simulink library "telem_conversion_lib"  (R2014b)
settings: Solver=ode45  StartTime=0.0  StopTime=10.0  RelTol=1e-3
undefined symbols (not defined in the file or in its folder): ini_moon_rotation_rate
libraries: util_quat_lib x11, util_frame_rotation_lib x4, util_common_lib x4, util_info_lib x1
settings Model: Creator=escrane  LastModifiedBy=mstewart

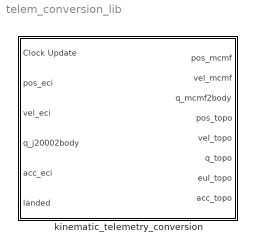
== system telem_conversion_lib ==
  kinematic_telemetry_conversion : Subsystem

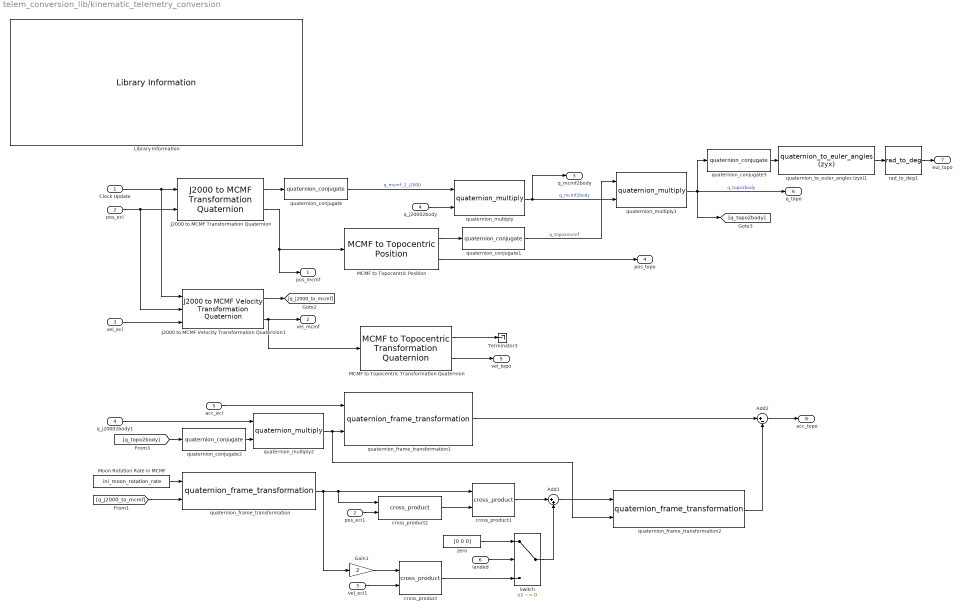
== system telem_conversion_lib/kinematic_telemetry_conversion ==
  Clock Update : Inport
  pos_eci : Inport  Port=2
  vel_eci : Inport  Port=3
  q_j20002body : Inport  Port=4
  acc_eci : Inport  Port=5
  landed : Inport  Port=6
  Add1 : Sum  Inputs=|++
  Add2 : Sum  Inputs=|+-
  Gain1 : Gain  Gain=2
  J2000 to MCMF Transformation Quaternion : util_frame_rotation_lib/J2000 to MCMF  Transformation Quaternion  SystemSampleTime=-1
  J2000 to MCMF Velocity Transformation Quaternion1 : util_frame_rotation_lib/J2000 to MCMF Velocity Transformation Quaternion  SystemSampleTime=-1
  Library Information : util_info_lib/Library Information  owner='NONE'
  MCMF to Topocentric Position : util_frame_rotation_lib/MCMF to Topocentric  Position  SystemSampleTime=-1
  MCMF to Topocentric Transformation Quaternion : util_frame_rotation_lib/MCMF to Topocentric  Transformation Quaternion  SystemSampleTime=-1
  Moon Rotation Rate in MCMF : Constant  Value=ini_moon_rotation_rate
  Switch : Switch  Criteria=u2 ~= 0
  Terminator3 : Terminator
  cross_product : util_common_lib/cross_product  SystemSampleTime=-1
  cross_product1 : util_common_lib/cross_product  SystemSampleTime=-1
  cross_product2 : util_common_lib/cross_product  SystemSampleTime=-1
  pos_eci1 : InportShadow  Port=2
  q_j20002body1 : InportShadow  Port=4
  quaternion_conjugate{,1..3} (4 alike) : util_quat_lib/quaternion_conjugate  SystemSampleTime=-1
  quaternion_frame_transformation : util_quat_lib/quaternion_frame_transformation  SystemSampleTime=-1
  quaternion_frame_transformation1 : util_quat_lib/quaternion_frame_transformation  SystemSampleTime=-1
  quaternion_frame_transformation2 : util_quat_lib/quaternion_frame_transformation  SystemSampleTime=-1
  quaternion_multiply : util_quat_lib/quaternion_multiply  SystemSampleTime=-1
  quaternion_multiply1 : util_quat_lib/quaternion_multiply  SystemSampleTime=-1
  quaternion_multiply2 : util_quat_lib/quaternion_multiply  SystemSampleTime=-1
  quaternion_to_euler_angles (zyx)1 : util_quat_lib/quaternion_to_euler_angles (zyx)  SystemSampleTime=-1
  rad_to_deg1 : util_common_lib/rad_to_deg  SystemSampleTime=-1
  vel_eci1 : InportShadow  Port=3
  zero : Constant  Value=[0 0 0]
  pos_mcmf : Outport
  vel_mcmf : Outport  Port=2
  q_mcmf2body : Outport  Port=3
  pos_topo : Outport  Port=4
  vel_topo : Outport  Port=5
  q_topo : Outport  Port=6
  eul_topo : Outport  Port=7
  acc_topo : Outport  Port=8
  wires:
  Switch/1 -> Add1/2
  zero/1 -> Switch/1
  landed/1 -> Switch/2
  J2000 to MCMF Transformation Quaternion/2 -> MCMF to Topocentric Position/1, pos_mcmf/1
  pos_eci/1 -> J2000 to MCMF Velocity Transformation Quaternion1/2, J2000 to MCMF Transformation Quaternion/2
  J2000 to MCMF Velocity Transformation Quaternion1/2 -> vel_mcmf/1, MCMF to Topocentric Transformation Quaternion/1
  MCMF to Topocentric Position/2 -> pos_topo/1
  MCMF to Topocentric Transformation Quaternion/1 -> Terminator3/1
  J2000 to MCMF Velocity Transformation Quaternion1/1 -> [q_j2000_to_mcmf]
  quaternion_multiply/1 -> quaternion_multiply1/2, q_mcmf2body/1  "q_mcmf2body"
  quaternion_multiply1/1 -> [q_topo2body], quaternion_conjugate3/1, q_topo/1  "q_topo2body"
  J2000 to MCMF Transformation Quaternion/1 -> quaternion_conjugate/1
  quaternion_conjugate/1 -> quaternion_multiply/1  "q_mcmf_2_j2000"
  q_j20002body/1 -> quaternion_multiply/2
  quaternion_conjugate1/1 -> quaternion_multiply1/1  "q_topo2mcmf"
  MCMF to Topocentric Position/1 -> quaternion_conjugate1/1
  MCMF to Topocentric Transformation Quaternion/2 -> vel_topo/1
  quaternion_to_euler_angles (zyx)1/1 -> rad_to_deg1/1
  rad_to_deg1/1 -> eul_topo/1
  vel_eci/1 -> J2000 to MCMF Velocity Transformation Quaternion1/3
  Clock Update/1 -> J2000 to MCMF Transformation Quaternion/1, J2000 to MCMF Velocity Transformation Quaternion1/1
  cross_product/1 -> Switch/3
  cross_product1/1 -> Add1/1
  pos_eci1/1 -> cross_product2/2
  cross_product2/1 -> cross_product1/2
  vel_eci1/1 -> cross_product/2
  Gain1/1 -> cross_product/1
  quaternion_frame_transformation/1 -> Gain1/1, cross_product1/1, cross_product2/1
  Moon Rotation Rate in MCMF/1 -> quaternion_frame_transformation/1
  [q_j2000_to_mcmf] -> quaternion_frame_transformation/2
  Add2/1 -> acc_topo/1
  q_j20002body1/1 -> quaternion_multiply2/1
  [q_topo2body] -> quaternion_conjugate2/1
  quaternion_conjugate2/1 -> quaternion_multiply2/2
  quaternion_multiply2/1 -> quaternion_frame_transformation2/2, quaternion_frame_transformation1/2
  acc_eci/1 -> quaternion_frame_transformation1/1
  quaternion_frame_transformation1/1 -> Add2/1
  quaternion_conjugate3/1 -> quaternion_to_euler_angles (zyx)1/1
  quaternion_frame_transformation2/1 -> Add2/2
  Add1/1 -> quaternion_frame_transformation2/1
